simulink model "Lab2"  (R2018a)
settings: Solver=VariableStepAuto  StartTime=0.0  StopTime=Time(end)  FixedStep=0.01  RelTol=1e-3
values from neighbouring files (symbols this model uses):
  Cf = Cf+1000    (= 21000)    [Init_for_washout_filter.m]
  Cr = Cr+1000    (= 31000)    [Init_for_washout_filter.m]
  lf = 0.41*2.55    (= 1.0455)    [Init_for_washout_filter.m]
  lr = 2.55-lf    (= 1.5045)    [Init_for_washout_filter.m]
  mass = 1435-80    (= 1355)    [Init_for_washout_filter.m]
  Ratio = 17    [Init_for_washout_filter.m]
  rollGrad = 5*(pi/180)    (= 0.0872664625997)    [Init_for_washout_filter.m]
  rx = 0.4    [Init_for_washout_filter.m]
  T = T+0.02    (= 0.42)    [Init_for_washout_filter.m]
settings Model: Creator=c_s  LastModifiedBy=c_s

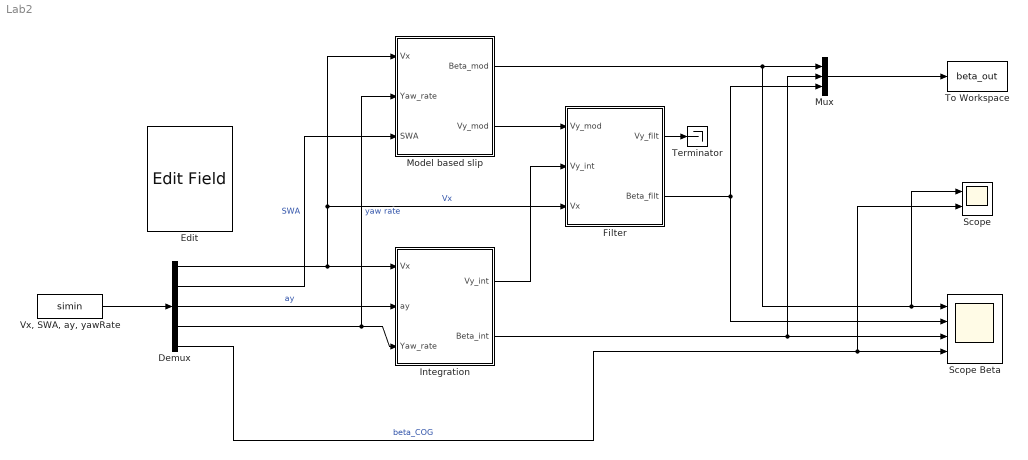
== system Lab2 ==
  Demux : Demux  Outputs=5
  Edit : EditField  Tag=T, filter constant  WebBlockId=163  Alignment=Center
  Filter : Subsystem
  Integration : Subsystem
  Model based slip : Subsystem
  Mux : Mux  Inputs=3
  Scope : Scope  NumInputPorts=2
  "Scope Beta " : Scope  NumInputPorts=4
  Terminator : Terminator
  To Workspace : ToWorkspace  VariableName=beta_out  SampleTime=-1
  "Vx, SWA, ay, yawRate" : FromWorkspace  VariableName=simin  SampleTime=0
  wires:
  "Vx, SWA, ay, yawRate"/1 -> Demux/1
  Model based slip/1(Beta_mod) -> Mux/1, Scope/1, "Scope Beta "/1
  Demux/1 -> Model based slip/1(Vx), Filter/3(Vx), Integration/1(Vx)  "Vx"
  Demux/2 -> Model based slip/3(SWA)  "SWA"
  Demux/3 -> Integration/2(ay)  "ay"
  Demux/4 -> Model based slip/2(Yaw_rate), Integration/3(Yaw_rate)  "yaw rate"
  Integration/1(Vy_int) -> Filter/2(Vy_int)
  Model based slip/2(Vy_mod) -> Filter/1(Vy_mod)
  Demux/5 -> Scope/2, "Scope Beta "/4  "beta_COG"
  Integration/2(Beta_int) -> Mux/2, "Scope Beta "/3
  Filter/2(Beta_filt) -> Mux/3, "Scope Beta "/2
  Mux/1 -> To Workspace/1
  Filter/1(Vy_filt) -> Terminator/1

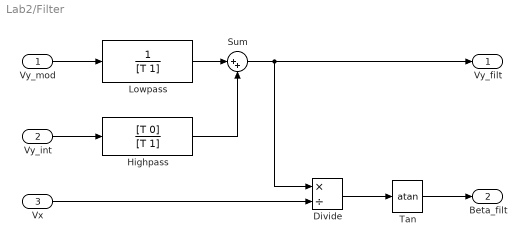
== system Lab2/Filter ==
  Vy_mod : Inport
  Vy_int : Inport  Port=2
  Vx : Inport  Port=3
  Divide : Product  Inputs=*/
  Highpass : TransferFcn  Numerator=[T 0]  Denominator=[T 1]
  Lowpass : TransferFcn  Denominator=[T 1]
  Sum : Sum  Inputs=|++
  Tan : Trigonometry  Operator=atan
  Vy_filt : Outport
  Beta_filt : Outport  Port=2
  wires:
  Vy_mod/1 -> Lowpass/1
  Vy_int/1 -> Highpass/1
  Lowpass/1 -> Sum/1
  Highpass/1 -> Sum/2
  Sum/1 -> Divide/1, Vy_filt/1
  Divide/1 -> Tan/1
  Tan/1 -> Beta_filt/1
  Vx/1 -> Divide/2

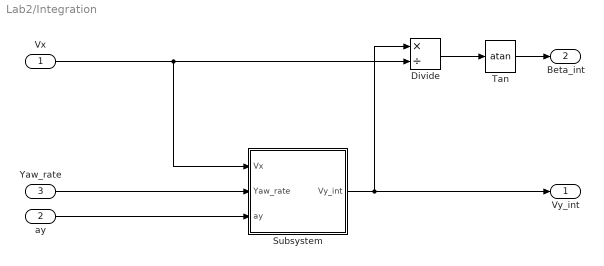
== system Lab2/Integration ==
  Vx : Inport
  ay : Inport  Port=2
  Yaw_rate : Inport  Port=3
  Divide : Product  Inputs=*/
  Subsystem : Subsystem
  Tan : Trigonometry  Operator=atan
  Vy_int : Outport
  Beta_int : Outport  Port=2
  wires:
  Vx/1 -> Subsystem/1(Vx), Divide/2
  Yaw_rate/1 -> Subsystem/2(Yaw_rate)
  ay/1 -> Subsystem/3(ay)
  Subsystem/1(Vy_int) -> Divide/1, Vy_int/1
  Divide/1 -> Tan/1
  Tan/1 -> Beta_int/1

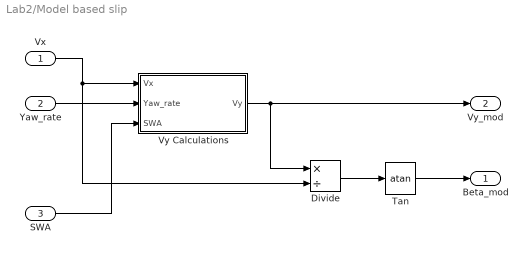
== system Lab2/Model based slip ==
  Vx : Inport
  Yaw_rate : Inport  Port=2
  SWA : Inport  Port=3
  Divide : Product  Inputs=*/
  Tan : Trigonometry  Operator=atan
  Vy Calculations : Subsystem
  Beta_mod : Outport
  Vy_mod : Outport  Port=2
  wires:
  Vx/1 -> Divide/2, Vy Calculations/1(Vx)
  Tan/1 -> Beta_mod/1
  Vy Calculations/1(Vy) -> Divide/1, Vy_mod/1
  Divide/1 -> Tan/1
  SWA/1 -> Vy Calculations/3(SWA)
  Yaw_rate/1 -> Vy Calculations/2(Yaw_rate)

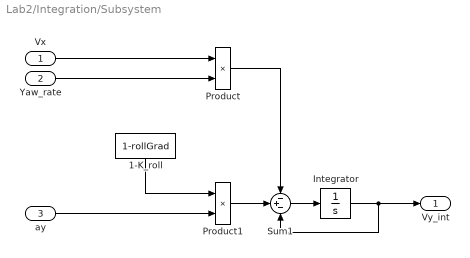
== system Lab2/Integration/Subsystem ==
  Vx : Inport
  Yaw_rate : Inport  Port=2
  ay : Inport  Port=3
  1-K_roll : Constant  Value=1-rollGrad
  Integrator : Integrator
  Product : Product
  Product1 : Product
  Sum1 : Sum  Inputs=-+-
  Vy_int : Outport
  wires:
  Product/1 -> Sum1/1
  Vx/1 -> Product/1
  Integrator/1 -> Sum1/3, Vy_int/1
  Yaw_rate/1 -> Product/2
  ay/1 -> Product1/2
  Product1/1 -> Sum1/2
  Sum1/1 -> Integrator/1
  1-K_roll/1 -> Product1/1

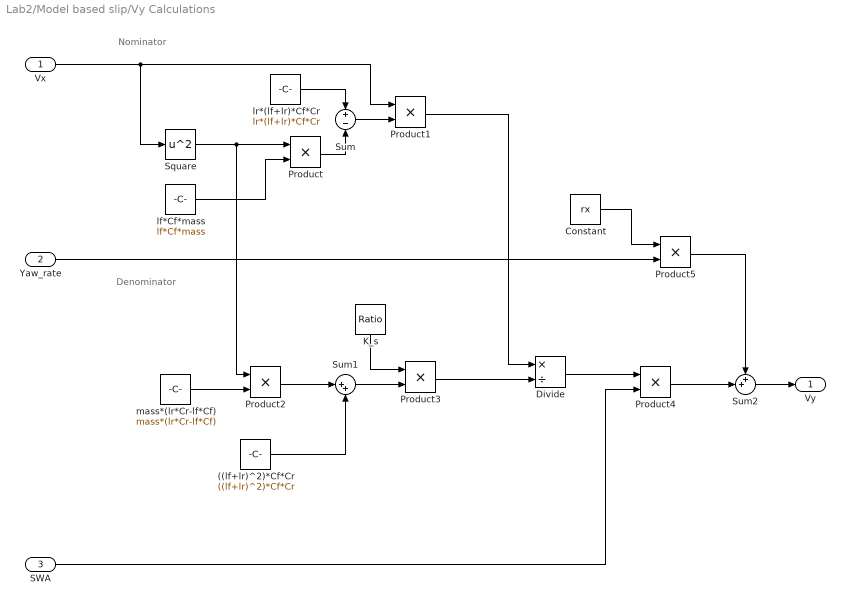
== system Lab2/Model based slip/Vy Calculations ==
  note: Nominator
  note: Denominator
  Vx : Inport
  Yaw_rate : Inport  Port=2
  SWA : Inport  Port=3
  ((lf+lr)^2)*Cf*Cr : Constant  Value=((lf+lr)^2)*Cf*Cr
  Constant : Constant  Value=rx
  Divide : Product  Inputs=*/
  K_s : Constant  Value=Ratio
  Product{,1..5} (6 alike) : Product
  Square : Math  Operator=square  RndMeth=Zero  SaturateOnIntegerOverflow=on
  Sum : Sum  Inputs=+-
  Sum1 : Sum  Inputs=|++
  Sum2 : Sum  Inputs=++|
  lf*Cf*mass : Constant  Value=lf*Cf*mass
  lr*(lf+lr)*Cf*Cr : Constant  Value=lr*(lf+lr)*Cf*Cr
  mass*(lr*Cr-lf*Cf) : Constant  Value=mass*(lr*Cr-lf*Cf)
  Vy : Outport
  wires:
  Product1/1 -> Divide/1
  Product3/1 -> Divide/2
  Vx/1 -> Product1/1, Square/1
  lr*(lf+lr)*Cf*Cr/1 -> Sum/1
  Sum/1 -> Product1/2
  Product/1 -> Sum/2
  Square/1 -> Product2/1, Product/1
  lf*Cf*mass/1 -> Product/2
  Product2/1 -> Sum1/1
  mass*(lr*Cr-lf*Cf)/1 -> Product2/2
  Sum1/1 -> Product3/2
  ((lf+lr)^2)*Cf*Cr/1 -> Sum1/2
  Divide/1 -> Product4/1
  SWA/1 -> Product4/2
  K_s/1 -> Product3/1
  Product4/1 -> Sum2/2
  Product5/1 -> Sum2/1
  Yaw_rate/1 -> Product5/2
  Constant/1 -> Product5/1
  Sum2/1 -> Vy/1
